simulink model "untitled1"  (R2018b)
settings: Solver=VariableStepAuto  StartTime=0.0  StopTime=10.0  RelTol=1e-3
libraries: simulink x1
settings Model: Creator=sn2xws  LastModifiedBy=sn2xws

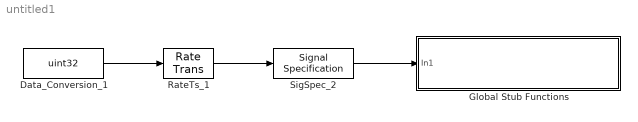
== system untitled1 ==
  Data_Conversion_1 : DataTypeConversion  OutDataTypeStr=uint32  SaturateOnIntegerOverflow=on  RndMeth=Zero
  Global Stub Functions : Subsystem  Tag=_SLT_SLFunc_Stub_
  RateTs_1 : RateTransition
  SigSpec_2 : SignalSpecification  OutDataTypeStr=uint32  Dimensions=[1]
  wires:
  ? -> Data_Conversion_1/1
  RateTs_1/1 -> SigSpec_2/1
  Data_Conversion_1/1 -> RateTs_1/1
  SigSpec_2/1 -> Global Stub Functions/1(In1)

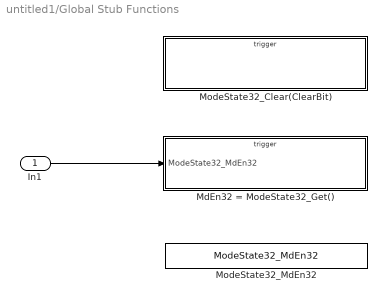
== system untitled1/Global Stub Functions ==
  In1 : Inport
  MdEn32 = ModeState32_Get() : Subsystem  Tag=_SLT_SLFunc_Stub_  TreatAsAtomicUnit=on
  ModeState32_Clear(ClearBit) : Subsystem  Tag=_SLT_SLFunc_Stub_  TreatAsAtomicUnit=on
  ModeState32_MdEn32 : DataStoreMemory  DataStoreName=ModeState32_MdEn32  ReadBeforeWriteMsg=warning  WriteAfterWriteMsg=warning  WriteAfterReadMsg=warning  ShowAdditionalParam=off  OutDataTypeStr=uint32  Dimensions=[1, 1]
  wires:
  In1/1 -> MdEn32 = ModeState32_Get()/1(ModeState32_MdEn32)

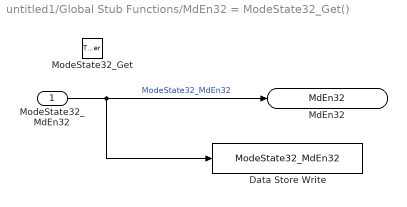
== system untitled1/Global Stub Functions/MdEn32 = ModeState32_Get() ==
  ModeState32_MdEn32 : Inport
  ModeState32_Get : TriggerPort  TriggerType=function-call  IsSimulinkFunction=on  FunctionName=ModeState32_Get  VariantControl=(inherit)
  Data Store Write : DataStoreWrite  DataStoreName=ModeState32_MdEn32
  MdEn32 : ArgOut  DisableCoverage=on  OutDataTypeStr=uint32  PortDimensions=[1, 1]  ArgumentName=MdEn32
  wires:
  ModeState32_MdEn32/1 -> Data Store Write/1, MdEn32/1  "ModeState32_MdEn32"

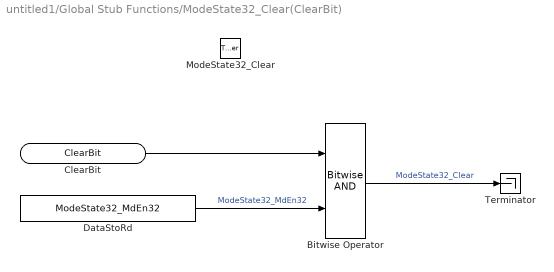
== system untitled1/Global Stub Functions/ModeState32_Clear(ClearBit) ==
  ModeState32_Clear : TriggerPort  TriggerType=function-call  IsSimulinkFunction=on  FunctionName=ModeState32_Clear  VariantControl=(inherit)
  Bitwise Operator : simulink/Logic and Bit Operations/Bitwise Operator  logicop=AND  UseBitMask=off  NumInputPorts=2  BitMask=bin2dec('11011001')  BitMaskRealWorld=Stored Integer
  DataStoRd : DataStoreRead  DataStoreName=ModeState32_MdEn32  DataStoreElements=ModeState32_MdEn32
  Terminator : Terminator
  ClearBit : ArgIn  DisableCoverage=on  OutDataTypeStr=uint32  PortDimensions=[1, 1]  ArgumentName=ClearBit
  wires:
  ClearBit/1 -> Bitwise Operator/1
  DataStoRd/1 -> Bitwise Operator/2  "ModeState32_MdEn32"
  Bitwise Operator/1 -> Terminator/1  "ModeState32_Clear"
